simulink model "PLL_Simulering"  (R2020a)
settings: Solver=VariableStepAuto  StartTime=0  StopTime=0.5  RelTol=1e-3
InitFcn:
  | clear all;
libraries: powerlib x48, eePowerMeasurement x1, powerlib_meascontrol x1
(part 1 of 3)
settings Model: OrderedModelArguments=off  Creator=Bausa  LastModifiedBy=Bausa
settings SolverCC: AlgebraicLoopSolver=LineSearch
settings DataIOCC: ReturnWorkspaceOutputsName=tp1bad6c91_55d6_49eb_9d82_9787064f6320
settings OptimizationCC: DefaultParameterBehavior=Inlined  EnhancedBackFolding=on  PassReuseOutputArgsAs=Individual arguments  ZeroExternalMemoryAtStartup=off  ZeroInternalMemoryAtStartup=off  OptimizeBlockOrder=speed  DifferentSizesBufferReuse=on  OptimizationCustomize=off  EfficientTunableParamExpr=on
settings DebuggingCC: ParameterTunabilityLossMsg=error
settings SFSimCC: SimCustomHeaderCode="#include \"C_Functions.h\""  SimUserSources=C_Functions.c  MATLABDynamicMemAlloc=off
settings RTWCC: SystemTargetFile=ert.tlc  TemplateMakefile=ert_default_tmf
settings CodeAppCC: ForceParamTrailComments=on  IgnoreCustomStorageClasses=off  OperatorAnnotations=on  SimulinkDataObjDesc=on  SFDataObjDesc=on  InsertBlockDesc=on
settings ERTTargetCC: TargetLangStandard=C99 (ISO)  GenerateSampleERTMain=on  InlinedParameterPlacement=NonHierarchical  ERTCustomFileTemplate=example_file_process.tlc

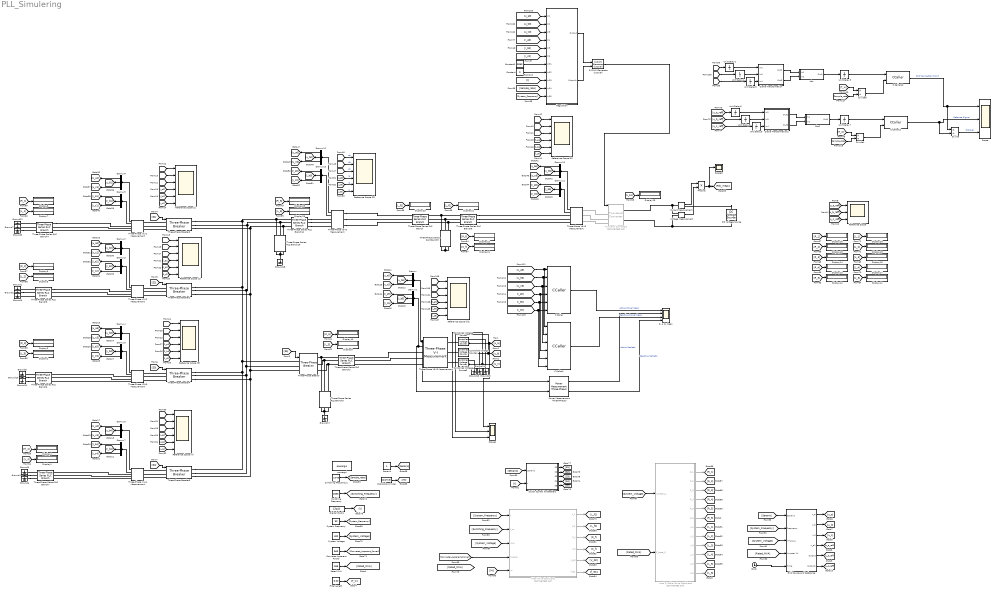
== system PLL_Simulering ==
  Abs : Subsystem
  Abs2 : Subsystem
  C Caller : CCaller  FunctionName=measure_P  PortSpecificationStruct="%)30     .    V L   8    (     @         %    \"     <    !     0         %  0 \"0    $    _    07)G3F%M90  4&]R=$YA;64 4V-O<&4     26YD97@     5'EP90      4VEZ90      27-';&]B86P   X    P    !@    @    $          4    (     0    ,    !         !   P!O=70 #@   #     &    \"     0         !0    @    !     P    $         $  # &]U=  .    .     8    (    !          %    \"     $    &     0         0   ...(+3703 chars)"
  C Caller1 : CCaller  FunctionName=measure_Q  PortSpecificationStruct="%)30     .    V L   8    (     @         %    \"     <    !     0         %  0 \"0    $    _    07)G3F%M90  4&]R=$YA;64 4V-O<&4     26YD97@     5'EP90      4VEZ90      27-';&]B86P   X    P    !@    @    $          4    (     0    ,    !         !   P!O=70 #@   #     &    \"     0         !0    @    !     P    $         $  # &]U=  .    .     8    (    !          %    \"     $    &     0         0   ...(+3703 chars)"
  C Caller10 : CCaller  FunctionName=MAF_Error_1  PortSpecificationStruct="%)30     .    : 4   8    (     @         %    \"     ,    !     0         %  0 \"0    $    _    07)G3F%M90  4&]R=$YA;64 4V-O<&4     26YD97@     5'EP90      4VEZ90      27-';&]B86P   X    P    !@    @    $          4    (     0    ,    !         !   P!O=70 #@   #     &    \"     0         !0    @    !     P    $         $  # &]U=  .    .     8    (    !          %    \"     $    &     0         0    !@   $]U='!U=   #@   #@    &    \"     8         !0    @    !     0    $         \"0    @               X    X    !@    @    $          4    (     0    8    !         !     &    9&]U8FQE   .    ,     8    (    !          %    \"     $    !     0         0  $ ,0    X    P    !@    @    ) @        4    (     0    $    !          (  0      #@   #@    &    \"     0         !0    @    !    !@    $         $     8   !S86UP;&4   X    X    !@    @    $          4    (     0    8    !         !     &    <V%M<&QE   .    .     8    (    !          %    \"     $    %     0         0    !0   $EN<'5T    #@   #@    &    \"     8         !0    @    !     0    $         \"0    @               X    X    !@    @    $          4    (     0    8    !         !     &    9&]U8FQE   .    ,     8    (    !          %    \"     $    !     0         0  $ ,0    X    P    !@    @    ) @        4    (     0    $    !          (  0      #@   #     &    \"     0         !0    @    !     P    $         $  # &QE;@ .    ,     8    (    !          %    \"     $    #     0         0  , ;&5N  X    X    !@    @    $          4    (     0    4    !         !     %    26YP=70    .    .     8    (    !@         %    \"     $    !     0         )    \"            / _#@   #@    &    \"     0         !0    @    !    !@    $         $     8   !U:6YT,S(   X    P    !@    @    $          4    (     0    $    !         !   0 Q    #@   #     &    \"     D\"        !0    @    !     0    $          @ !"
  C Caller12 : CCaller  FunctionName=MAF_Error_2  PortSpecificationStruct="%)30     .    : 4   8    (     @         %    \"     ,    !     0         %  0 \"0    $    _    07)G3F%M90  4&]R=$YA;64 4V-O<&4     26YD97@     5'EP90      4VEZ90      27-';&]B86P   X    P    !@    @    $          4    (     0    ,    !         !   P!O=70 #@   #     &    \"     0         !0    @    !     P    $         $  # &]U=  .    .     8    (    !          %    \"     $    &     0         0    !@   $]U='!U=   #@   #@    &    \"     8         !0    @    !     0    $         \"0    @               X    X    !@    @    $          4    (     0    8    !         !     &    9&]U8FQE   .    ,     8    (    !          %    \"     $    !     0         0  $ ,0    X    P    !@    @    ) @        4    (     0    $    !          (  0      #@   #@    &    \"     0         !0    @    !    !@    $         $     8   !S86UP;&4   X    X    !@    @    $          4    (     0    8    !         !     &    <V%M<&QE   .    .     8    (    !          %    \"     $    %     0         0    !0   $EN<'5T    #@   #@    &    \"     8         !0    @    !     0    $         \"0    @               X    X    !@    @    $          4    (     0    8    !         !     &    9&]U8FQE   .    ,     8    (    !          %    \"     $    !     0         0  $ ,0    X    P    !@    @    ) @        4    (     0    $    !          (  0      #@   #     &    \"     0         !0    @    !     P    $         $  # &QE;@ .    ,     8    (    !          %    \"     $    #     0         0  , ;&5N  X    X    !@    @    $          4    (     0    4    !         !     %    26YP=70    .    .     8    (    !@         %    \"     $    !     0         )    \"            / _#@   #@    &    \"     0         !0    @    !    !@    $         $     8   !U:6YT,S(   X    P    !@    @    $          4    (     0    $    !         !   0 Q    #@   #     &    \"     D\"        !0    @    !     0    $          @ !"
  Clarke Transformation : Subsystem
  Clarke Transformation2 : Subsystem
  Clock : Clock
  Constant : Constant  Value=0
  Constant1 : Constant  Value=50e3
  Controlled Voltage Source : powerlib/Electrical Sources/Controlled Voltage Source  Initialize=off  Source_Type=AC  Amplitude=0  Phase=0  Frequency=0  Measurements=None
  Controlled Voltage Source1 : powerlib/Electrical Sources/Controlled Voltage Source  Initialize=off  Source_Type=AC  Amplitude=0  Phase=0  Frequency=0  Measurements=None
  Controlled Voltage Source2 : powerlib/Electrical Sources/Controlled Voltage Source  Initialize=off  Source_Type=AC  Amplitude=0  Phase=0  Frequency=0  Measurements=None
  Converter Apparent Power : Constant  Value=5e3
  Current Measurement : powerlib/Measurements/Current Measurement  PhasorSimulation=off  OutputType=Complex  PSBequivalent=0
  DC Voltage Source : powerlib/Electrical Sources/DC Voltage Source  Amplitude=400  Measurements=None
  Demux{,1..13} (14 alike) : Demux  Outputs=3
  Digital Clock1 : DigitalClock
  Display{1..25,28..29} (27 alike) : Display
      Display1 settings: Format=short_e
      Display21 settings: Format=short_e
      Display23 settings: Format=short_e
      Display24 settings: Format=short_e
      Display25 settings: Format=short_e
      Display29 settings: Format=short_e
      Display5 settings: Format=short_e
      Display7 settings: Format=short_e
      Display9 settings: Format=short_e
  Divide : Product  Inputs=*/
  Divide1 : Product  Inputs=*/  OutDataTypeStr=uint32
  Divide3 : Product  Inputs=*/  OutDataTypeStr=uint32
  Filter Length : Constant  Value=0.02
  Filter Value Coeficients : MATLAB Function  Commented=on  TreatAsAtomicUnit=on
  Grid Source and Referance : Subsystem
  Ground{1..15,17..18} (17 alike) : powerlib/Elements/Ground  LConnTagsString=a
  Load & Cable Value Coeficients : MATLAB Function  Commented=on  TreatAsAtomicUnit=on
  Modulations Index : Constant  Value=2/sqrt(3)
  P- & Q- Meas. : Scope  NumInputPorts=4
  Power Measurement (Three-Phase) : eePowerMeasurement/Power Measurement (Three-Phase)  LabelModeActiveChoice=Continuous  F=60  K=[0]  Seq=Positive  Ts=0
      settings: SourceProductBaseCode=PS
  Product : Product
  Rated MVA : Constant  Value=2e6
  Referance Scope : Scope  NumInputPorts=3
  Referance Scope [0] : Scope  NumInputPorts=6
  Referance Scope [0]1 : Scope  NumInputPorts=6
  Referance Scope [1] : Scope  NumInputPorts=6
  Referance Scope [2] : Scope  NumInputPorts=6
  Referance Scope [3] : Scope  NumInputPorts=6
  Referance Scope [4] : Scope  NumInputPorts=6
  Referance Scope [6] : Scope  NumInputPorts=6
  Regulation : Subsystem
  SVPWM Generator (2-Level) : powerlib_meascontrol/Pulse & Signal Generators/SVPWM Generator (2-Level)  InputType=alpha-beta components  SwitchingPattern=Pattern #1  Fc=3000  ParUref=[0.8 0 50]  Ts=1e-6
      settings: SourceProductBaseCode=PS
  Scope : Scope  NumInputPorts=3
  Scope1 : Scope  NumInputPorts=3
  Scope3 : Scope
  Senario : Constant
  Switch Control for Breakers : MATLAB Function  TreatAsAtomicUnit=on
  Switching Frequency : Constant  Value=15e3
  Switching Frequency2 : Constant  Value=1e-06  OutDataTypeStr=double
  System Frequency : Constant  Value=50
  System Voltage : Constant  Value=400
  Three-Phase Series RLC Branch : powerlib/Elements/Three-Phase Series RLC Branch  LConnTagsString=A|B|C  RConnTagsString=A|B|C  BranchType=L  Resistance=1  Inductance=1.8e-3  Capacitance=1e-6  Measurements=None
  Three-Phase Series RLC Branch10 : powerlib/Elements/Three-Phase Series RLC Branch  LConnTagsString=A|B|C  RConnTagsString=A|B|C  BranchType=R  Resistance=1e9  Inductance=1e-3  Capacitance=1e-6  Measurements=None
  Three-Phase Series RLC Branch11 : powerlib/Elements/Three-Phase Series RLC Branch  LConnTagsString=A|B|C  RConnTagsString=A|B|C  BranchType=RL  Resistance=0.008268  Inductance=7.9572e-2  Capacitance=1e-6  Measurements=None
  Three-Phase Series RLC Branch2 : powerlib/Elements/Three-Phase Series RLC Branch  LConnTagsString=A|B|C  RConnTagsString=A|B|C  BranchType=RL  Resistance=0.005968  Inductance=1.9e-5  Capacitance=1e-6  Measurements=None
  Three-Phase Series RLC Branch3 : powerlib/Elements/Three-Phase Series RLC Branch  LConnTagsString=A|B|C  RConnTagsString=A|B|C  BranchType=R  Resistance=1e9  Inductance=1e-3  Capacitance=1e-6  Measurements=None
  Three-Phase Series RLC Branch{4..7} (4 alike) : powerlib/Elements/Three-Phase Series RLC Branch  LConnTagsString=A|B|C  RConnTagsString=A|B|C  BranchType=RL  Resistance=0.005968  Inductance=1.9e-4  Capacitance=1e-6  Measurements=None
  Three-Phase Series RLC Branch8 : powerlib/Elements/Three-Phase Series RLC Branch  LConnTagsString=A|B|C  RConnTagsString=A|B|C  BranchType=L  Resistance=1  Inductance=3e-4  Capacitance=1e-6  Measurements=None
  Three-Phase Series RLC Branch9 : powerlib/Elements/Three-Phase Series RLC Branch  LConnTagsString=A|B|C  RConnTagsString=A|B|C  BranchType=RC  Resistance=1e-6  Inductance=1e-3  Capacitance=25e-3  Measurements=None
  Three-Phase V0-I0 Measurement : powerlib/Measurements/Three-Phase V-I Measurement  VoltageMeasurement=phase-to-ground  SetLabelV=off  LabelV=Vabc  Vpu=off  VpuLL=off  CurrentMeasurement=yes  SetLabelI=off  LabelI=Iabc  Ipu=off  Pbase=100e6  Vbase=500e3  OutputType=Complex  PhasorSimulation=off  PSBequivalent=0
  Three-Phase V1-I1 Measurement : powerlib/Measurements/Three-Phase V-I Measurement  VoltageMeasurement=phase-to-ground  SetLabelV=off  LabelV=Vabc  Vpu=off  VpuLL=off  CurrentMeasurement=yes  SetLabelI=off  LabelI=Iabc  Ipu=off  Pbase=100e6  Vbase=500e3  OutputType=Complex  PhasorSimulation=off  PSBequivalent=0
  Three-Phase V2-I2 Measurement : powerlib/Measurements/Three-Phase V-I Measurement  VoltageMeasurement=phase-to-ground  SetLabelV=off  LabelV=Vabc  Vpu=off  VpuLL=off  CurrentMeasurement=yes  SetLabelI=off  LabelI=Iabc  Ipu=off  Pbase=100e6  Vbase=500e3  OutputType=Complex  PhasorSimulation=off  PSBequivalent=0
  Three-Phase V3-I3 Measurement : powerlib/Measurements/Three-Phase V-I Measurement  VoltageMeasurement=phase-to-ground  SetLabelV=off  LabelV=Vabc  Vpu=off  VpuLL=off  CurrentMeasurement=yes  SetLabelI=off  LabelI=Iabc  Ipu=off  Pbase=100e6  Vbase=500e3  OutputType=Complex  PhasorSimulation=off  PSBequivalent=0
  Three-Phase V4-I4 Measurement : powerlib/Measurements/Three-Phase V-I Measurement  VoltageMeasurement=phase-to-ground  SetLabelV=off  LabelV=Vabc  Vpu=off  VpuLL=off  CurrentMeasurement=yes  SetLabelI=off  LabelI=Iabc  Ipu=off  Pbase=100e6  Vbase=500e3  OutputType=Complex  PhasorSimulation=off  PSBequivalent=0
  Three-Phase V5-I5 Measurement : powerlib/Measurements/Three-Phase V-I Measurement  VoltageMeasurement=phase-to-ground  SetLabelV=off  LabelV=Vabc  Vpu=off  VpuLL=off  CurrentMeasurement=yes  SetLabelI=off  LabelI=Iabc  Ipu=off  Pbase=100e6  Vbase=500e3  OutputType=Complex  PhasorSimulation=off  PSBequivalent=0
  Three-Phase V6-I6 Measurement : powerlib/Measurements/Three-Phase V-I Measurement  VoltageMeasurement=phase-to-ground  SetLabelV=off  LabelV=Vabc  Vpu=off  VpuLL=off  CurrentMeasurement=yes  SetLabelI=off  LabelI=Iabc  Ipu=off  Pbase=100e6  Vbase=500e3  OutputType=Complex  PhasorSimulation=off  PSBequivalent=0
  Three-Phase Breaker : powerlib/Elements/Three-Phase Breaker  InitialState=open  SwitchA=on  SwitchB=on  SwitchC=on  SwitchTimes=9999  External=on  BreakerResistance=0.00001  SnubberResistance=1e9  SnubberCapacitance=0  Measurements=None
  Three-Phase Breaker{1..4} (4 alike) : powerlib/Elements/Three-Phase Breaker  InitialState=open  SwitchA=on  SwitchB=on  SwitchC=on  SwitchTimes="[1/60  5/60]"  External=on  BreakerResistance=0.01  SnubberResistance=1e6  SnubberCapacitance=inf  Measurements=None
  Two-Level Converter1 : powerlib/Power Electronics/Two-Level Converter  Commented=on  ModelType=Switching devices  Ron=1e-6  Rs=1e6  Cs=inf  Vforward=[0,0]  Ron_Diode=1e-3  Rs_Diode=1e6  Cs_Diode=inf  Vf_Diode=1e-3  Rs_CurrentSource=inf
      settings: SourceProductBaseCode=PS
  Unit Delay{2..9} (8 alike) : UnitDelay  SampleTime=-1  HasFrameUpgradeWarning=on
  Voltage Measurement : powerlib/Measurements/Voltage Measurement  PhasorSimulation=off  OutputType=Complex  PSBequivalent=0
  powergui : powerlib/powergui  Priority=1  SimulationMode=Discrete  SampleTime=1e-6  frequency=60  Iterations=50  frequencyindice=0  Pbase=100e6  ErrMax=1e-4  UnitsV=kV  UnitsW=MW  buscounter=0  FunctionMessages=off  echomessages=off  EnableUseOfTLC=off  CurrentSourceSwitches=off  DisableSnubberDevices=off  DisableRonSwitches=off  DisableVfSwitches=off  DisplayEquations=off  AutomaticDiscreteSolvers=off  SolverType=Tustin/Backward Euler (TBE)  Interpol=off  ExternalGateDelay=off  methode=off  Ts=100  x0status=blocks  SPID=on  SwTol=0  HookPort=off  NonlinearTolerance=1e-4  nMaxIteration=100  ContinueOnMaxIteration=off  RestoreLinks=warning  ResistiveCurrentMeasurement=off  Frange=[0:2:500]  Ylog=off  Xlog=on  ShowGrid=off  save=off  variable=ZData  structure=0  ZoomFFT=off  StartTime=0.0  cycles=1  DisplayStyle=1  fundamental=60  FreqAxis=off  MaxFrequency=1000  frequencyindicesteady=1  RmsSteady=1  display=off
  wires:
  Grid Source and Referance/1(u_a) -> [u_a]
  Grid Source and Referance/2(u_b) -> [u_b]
  Grid Source and Referance/3(u_c) -> [u_c]
  [u_a] -> Controlled Voltage Source/1, Scope1/1
  [u_c] -> Scope1/3, Controlled Voltage Source2/1
  [u_b] -> Scope1/2, Controlled Voltage Source1/1
  [S1] -> Three-Phase Breaker2/1
  [S2] -> Three-Phase Breaker1/1
  [S3] -> Three-Phase Breaker4/1
  [S4] -> Three-Phase Breaker3/1
  Three-Phase V5-I5 Measurement/1 -> Power Measurement (Three-Phase)/1, Demux/1
  Three-Phase V5-I5 Measurement/2 -> Power Measurement (Three-Phase)/2, Demux1/1
  [u_a_reff] -> Referance Scope/1
  [u_b_reff] -> Referance Scope/2
  [u_c_reff] -> Referance Scope/3
  Demux/1 -> [u_a5]
  Demux/2 -> [u_b5]
  Demux/3 -> [u_c5]
  Demux1/3 -> [i_c5]
  Demux1/1 -> [i_a5]
  Demux1/2 -> [i_b5]
  Demux6/1 -> [u_a4]
  Demux7/1 -> [i_a4]
  Demux7/3 -> [i_c4]
  Demux7/2 -> [i_b4]
  Demux6/2 -> [u_b4]
  Three-Phase V4-I4 Measurement/1 -> Demux6/1
  Demux6/3 -> [u_c4]
  Three-Phase V4-I4 Measurement/2 -> Demux7/1
  Demux4/1 -> [u_a3]
  Demux5/1 -> [i_a3]
  Demux5/3 -> [i_c3]
  Demux5/2 -> [i_b3]
  Demux4/2 -> [u_b3]
  Three-Phase V3-I3 Measurement/1 -> Demux4/1
  Demux4/3 -> [u_c3]
  Three-Phase V3-I3 Measurement/2 -> Demux5/1
  Demux2/1 -> [u_a2]
  Demux3/1 -> [i_a2]
  Demux3/3 -> [i_c2]
  Demux3/2 -> [i_b2]
  Demux2/2 -> [u_b2]
  Three-Phase V2-I2 Measurement/1 -> Demux2/1
  Demux2/3 -> [u_c2]
  Three-Phase V2-I2 Measurement/2 -> Demux3/1
  Demux8/1 -> [u_a1]
  Demux9/1 -> [i_a1]
  Demux9/3 -> [i_c1]
  Demux9/2 -> [i_b1]
  Demux8/2 -> [u_b1]
  Three-Phase V1-I1 Measurement/1 -> Demux8/1
  Demux8/3 -> [u_c1]
  Three-Phase V1-I1 Measurement/2 -> Demux9/1
  Demux10/2 -> [u_b6]
  Demux10/1 -> [u_a6]
  Demux11/1 -> [i_a6]
  Demux11/2 -> [i_b6]
  Demux11/3 -> [i_c6]
  Three-Phase V6-I6 Measurement/2 -> Demux11/1
  Demux10/3 -> [u_c6]
  Three-Phase V6-I6 Measurement/1 -> Demux10/1
  [u_c1] -> Referance Scope [1]/3
  [u_b1] -> Referance Scope [1]/2
  [u_a1] -> Referance Scope [1]/1
  [i_a1] -> Referance Scope [1]/4
  [i_b1] -> Referance Scope [1]/5
  [i_c1] -> Referance Scope [1]/6
  [i_b2] -> Referance Scope [2]/5
  [i_a2] -> Referance Scope [2]/4
  [i_c2] -> Referance Scope [2]/6
  [u_b2] -> Referance Scope [2]/2
  [u_c2] -> Referance Scope [2]/3
  [u_a2] -> Referance Scope [2]/1
  [i_b3] -> Referance Scope [3]/5
  [i_a3] -> Referance Scope [3]/4
  [i_c3] -> Referance Scope [3]/6
  [u_b3] -> Referance Scope [3]/2
  [u_c3] -> Referance Scope [3]/3
  [u_a3] -> Referance Scope [3]/1
  [i_b4] -> Referance Scope [4]/5
  [i_a4] -> Referance Scope [4]/4
  [i_c4] -> Referance Scope [4]/6
  [u_b4] -> Referance Scope [4]/2
  [u_c4] -> Referance Scope [4]/3
  [u_a4] -> Referance Scope [4]/1
  [i_b6] -> Referance Scope [6]/5
  [i_a6] -> Referance Scope [6]/4
  [i_c6] -> Referance Scope [6]/6
  [u_b6] -> Referance Scope [6]/2
  [u_c6] -> Referance Scope [6]/3
  [u_a6] -> Referance Scope [6]/1
  Demux12/2 -> [u_b0]
  Demux13/3 -> [i_c0]
  Demux12/3 -> [u_c0]
  Demux12/1 -> [u_a0]
  Demux13/1 -> [i_a0]
  Demux13/2 -> [i_b0]
  Three-Phase V0-I0 Measurement/1 -> Demux12/1
  Three-Phase V0-I0 Measurement/2 -> Demux13/1
  [u_b0] -> Referance Scope [0]/2  "Ub"
  [u_c0] -> Referance Scope [0]/3  "Uc"
  [i_c0] -> Referance Scope [0]/6  "Ic"
  [u_a0] -> Referance Scope [0]/1  "Ua"
  [i_a0] -> Referance Scope [0]/4  "Ia"
  [i_b0] -> Referance Scope [0]/5  "Ib"
  Grid Source and Referance/6(Output1) -> [u_c_reff]
  Grid Source and Referance/5(Output) -> [u_b_reff]
  Grid Source and Referance/4(u_a1) -> [u_a_reff]
  [R_4] -> Display4/1
  [L_4] -> Display1/1
  [R_3] -> Display3/1
  [L_3] -> Display2/1
  [R_2] -> Display6/1
  [L_2] -> Display5/1
  [R_1] -> Display8/1
  [L_1] -> Display7/1
  [R_5] -> Display10/1
  [L_5] -> Display9/1
  [R_5] -> Display12/1
  [R_3] -> Display14/1
  [R_4] -> Display13/1
  [R_1] -> Display16/1
  [R_2] -> Display15/1
  [L_4] -> Display17/1
  [L_3] -> Display18/1
  [L_1] -> Display20/1
  [L_2] -> Display19/1
  [L_5] -> Display11/1
  Divide/1 -> Scope/3  "Risidual"
  SVPWM Generator (2-Level)/1 -> Two-Level Converter1/1
  Switching Frequency/1 -> [Switching_Frequency]
  System Voltage/1 -> [System_Voltage]
  Senario/1 -> [Senario]
  Converter Apparent Power/1 -> [Converter_Apparent_Power]
  System Frequency/1 -> [System_Frequency]
  Switch Control for Breakers/1(S1) -> [S1]
  Switch Control for Breakers/5(S5) -> [S5]
  Switch Control for Breakers/2(S2) -> [S2]
  [t] -> Switch Control for Breakers/2(t)
  Switch Control for Breakers/3(S3) -> [S3]
  Switch Control for Breakers/4(S4) -> [S4]
  [Senario] -> Switch Control for Breakers/1(senario)
  Digital Clock1/1 -> [t]
  [System_Frequency] -> Filter Value Coeficients/1(f)
  [Switching_Frequency] -> Filter Value Coeficients/2(f_sw)
  Filter Value Coeficients/2(L_2) -> [L_f2]
  Filter Value Coeficients/1(L_1) -> [L_f1]
  Filter Value Coeficients/6(f_res) -> [f_res]
  [Mi] -> Filter Value Coeficients/5(Mi)
  Filter Value Coeficients/5(V_DC) -> [V_DC]
  Filter Value Coeficients/3(R_f) -> [R_f]
  [System_Voltage] -> Filter Value Coeficients/3(U_LL)
  Filter Value Coeficients/4(C_f) -> [C_f]
  Modulations Index/1 -> [Mi]
  Load & Cable Value Coeficients/3(R_3) -> [R_3]
  Load & Cable Value Coeficients/2(R_2) -> [R_2]
  Load & Cable Value Coeficients/4(R_4) -> [R_4]
  [System_Voltage] -> Load & Cable Value Coeficients/1(V_base_LL)
  Load & Cable Value Coeficients/11(L_5) -> [L_5]
  Load & Cable Value Coeficients/10(L_4) -> [L_4]
  Load & Cable Value Coeficients/9(L_3) -> [L_3]
  [Rated_MVA] -> Load & Cable Value Coeficients/2(S_base_3)
  Load & Cable Value Coeficients/8(L_2) -> [L_2]
  Load & Cable Value Coeficients/5(R_5) -> [R_5]
  Load & Cable Value Coeficients/7(L_1) -> [L_1]
  Load & Cable Value Coeficients/1(R_1) -> [R_1]
  Clock/1 -> Grid Source and Referance/5(Time)
  [Rated_MVA] -> Grid Source and Referance/4(Inverter VA)
  [System_Voltage] -> Grid Source and Referance/3(init_U_LL)
  [System_Frequency] -> Grid Source and Referance/2(Frequency)
  [Senario] -> Grid Source and Referance/1(Senario)
  [R_f] -> Display22/1
  [L_f1] -> Display21/1
  [L_f2] -> Display23/1
  [C_f] -> Display24/1
  [V_DC] -> Display25/1
  Rated MVA/1 -> [Rated_MVA]
  Load & Cable Value Coeficients/6(R_6) -> [R_6]
  Load & Cable Value Coeficients/12(L_6) -> [L_6]
  [i_a5] -> Referance Scope [0]1/4
  [i_b5] -> Referance Scope [0]1/5
  [i_c5] -> Referance Scope [0]1/6
  [u_a5] -> Referance Scope [0]1/1
  [u_b5] -> Referance Scope [0]1/2
  [u_c5] -> Referance Scope [0]1/3
  Clarke Transformation/1(Out2) -> Abs/1(In1)
  Clarke Transformation/2(Out3) -> Abs/2(In2)
  Filter Length/1 -> [T_w]
  Switching Frequency2/1 -> [Sample_rate]
  [Sample_rate] -> Divide3/2
  [T_w] -> Divide3/1
  C Caller10/1 -> Scope/1, Divide/1  "Grid Connection Point"
  Divide3/1 -> C Caller10/2
  Unit Delay3/1 -> C Caller10/1
  Abs/1(Out1) -> Unit Delay3/1
  [u_a0] -> Unit Delay2/1
  Unit Delay2/1 -> Clarke Transformation/1(In2)
  [u_b0] -> Unit Delay4/1
  Unit Delay4/1 -> Clarke Transformation/2(In3)
  Unit Delay5/1 -> Clarke Transformation/3(In4)
  [u_c0] -> Unit Delay5/1
  [u_b_reff] -> Unit Delay8/1
  Abs2/1(Out1) -> Unit Delay7/1
  [u_a_reff] -> Unit Delay6/1
  Unit Delay8/1 -> Clarke Transformation2/2(In3)
  Divide1/1 -> C Caller12/2
  Clarke Transformation2/2(Out3) -> Abs2/2(In2)
  C Caller12/1 -> Divide/2, Scope/2  "Refrance Signal"
  [T_w] -> Divide1/1
  [u_c_reff] -> Unit Delay9/1
  [Sample_rate] -> Divide1/2
  Unit Delay6/1 -> Clarke Transformation2/1(In2)
  Unit Delay9/1 -> Clarke Transformation2/3(In4)
  Clarke Transformation2/1(Out2) -> Abs2/1(In1)
  Unit Delay7/1 -> C Caller12/1
  [R_6] -> Display28/1
  [L_6] -> Display29/1
  [Converter_Apparent_Power] -> Filter Value Coeficients/4(S_base)
  Current Measurement/1 -> Product/1
  Voltage Measurement/1 -> Product/2
  Product/1 -> Scope3/1, [Pdc_meas]
  [S5] -> Three-Phase Breaker/1
  [Sample_rate] -> Regulation/10(In34)
  Constant/1 -> Regulation/8(In32)
  Constant1/1 -> Regulation/7(In31)
  [i_c0] -> Regulation/6(In6)
  [i_b0] -> Regulation/5(In5)
  [u_c0] -> Regulation/3(In3)
  [u_a0] -> Regulation/1(In1)
  Regulation/1(Output) -> SVPWM Generator (2-Level)/1
  Regulation/2(Output1) -> SVPWM Generator (2-Level)/2
  [t] -> Regulation/9(In33)
  [System_Frequency] -> Regulation/11(In35)
  [i_a0] -> Regulation/4(In4)
  [u_b0] -> Regulation/2(In2)
  [u_a5] -> C Caller1/1, C Caller/1
  [u_b5] -> C Caller1/2, C Caller/2
  [u_c5] -> C Caller1/3, C Caller/3
  [i_a5] -> C Caller1/4, C Caller/4
  [i_b5] -> C Caller1/5, C Caller/5
  [i_c5] -> C Caller1/6, C Caller/6
  C Caller/1 -> P- & Q- Meas./1  "Active Power Meas."
  C Caller1/1 -> P- & Q- Meas./3  "Reactive Power Meas."
  Power Measurement (Three-Phase)/1 -> P- & Q- Meas./2  "Active Matlabs"
  Power Measurement (Three-Phase)/2 -> P- & Q- Meas./4  "Reactive Matlabs"
  connections:
  Controlled Voltage Source/RConn1 -- Three-Phase V5-I5 Measurement/LConn1
  Controlled Voltage Source1/RConn1 -- Three-Phase V5-I5 Measurement/LConn2
  Controlled Voltage Source2/RConn1 -- Three-Phase V5-I5 Measurement/LConn3
  Three-Phase Breaker4/RConn1 -- Three-Phase Breaker3/RConn1 -- Three-Phase Series RLC Branch10/LConn1 -- Three-Phase Series RLC Branch11/LConn1 -- Three-Phase Breaker2/RConn1 -- Three-Phase Breaker1/RConn1 -- Three-Phase Breaker/LConn1
  DC Voltage Source/LConn1 -- Voltage Measurement/LConn2 -- Two-Level Converter1/RConn2
  Three-Phase Breaker2/LConn3 -- Three-Phase V1-I1 Measurement/LConn3
  Three-Phase Series RLC Branch4/RConn1 -- Three-Phase V1-I1 Measurement/RConn1
  Three-Phase V1-I1 Measurement/RConn3 -- Three-Phase Series RLC Branch4/RConn3
  Three-Phase Breaker2/LConn1 -- Three-Phase V1-I1 Measurement/LConn1
  Three-Phase Breaker2/LConn2 -- Three-Phase V1-I1 Measurement/LConn2
  Three-Phase V0-I0 Measurement/LConn3 -- Three-Phase Series RLC Branch/LConn3
  Two-Level Converter1/LConn1 -- Three-Phase V6-I6 Measurement/LConn1
  Two-Level Converter1/LConn2 -- Three-Phase V6-I6 Measurement/LConn2
  Three-Phase Series RLC Branch4/LConn1 -- Ground12/LConn1
  Ground8/LConn1 -- Three-Phase Series RLC Branch4/LConn3
  Two-Level Converter1/LConn3 -- Three-Phase V6-I6 Measurement/LConn3
  Three-Phase Breaker1/LConn1 -- Three-Phase V2-I2 Measurement/LConn1
  Three-Phase Breaker1/LConn3 -- Three-Phase V2-I2 Measurement/LConn3
  Three-Phase Breaker1/LConn2 -- Three-Phase V2-I2 Measurement/LConn2
  Three-Phase Breaker4/LConn1 -- Three-Phase V3-I3 Measurement/LConn1
  Three-Phase Breaker4/LConn2 -- Three-Phase V3-I3 Measurement/LConn2
  Three-Phase Breaker4/LConn3 -- Three-Phase V3-I3 Measurement/LConn3
  Three-Phase Breaker3/LConn3 -- Three-Phase V4-I4 Measurement/LConn3
  Three-Phase Breaker3/LConn1 -- Three-Phase V4-I4 Measurement/LConn1
  Three-Phase Breaker3/LConn2 -- Three-Phase V4-I4 Measurement/LConn2
  Ground15/LConn1 -- Controlled Voltage Source/LConn1
  Ground14/LConn1 -- Controlled Voltage Source1/LConn1
  Ground13/LConn1 -- Controlled Voltage Source2/LConn1
  Three-Phase Breaker4/RConn2 -- Three-Phase Breaker3/RConn2 -- Three-Phase Series RLC Branch10/LConn2 -- Three-Phase Series RLC Branch11/LConn2 -- Three-Phase Breaker2/RConn2 -- Three-Phase Breaker1/RConn2 -- Three-Phase Breaker/LConn2
  Three-Phase Breaker4/RConn3 -- Three-Phase Breaker3/RConn3 -- Three-Phase Breaker/LConn3 -- Three-Phase Series RLC Branch11/LConn3 -- Three-Phase Series RLC Branch10/LConn3 -- Three-Phase Breaker2/RConn3 -- Three-Phase Breaker1/RConn3
  Three-Phase Series RLC Branch2/LConn3 -- Three-Phase Series RLC Branch3/LConn3 -- Three-Phase Breaker/RConn3
  Three-Phase Series RLC Branch5/LConn3 -- Ground3/LConn1
  Three-Phase V2-I2 Measurement/RConn3 -- Three-Phase Series RLC Branch5/RConn3
  Three-Phase Series RLC Branch5/LConn1 -- Ground1/LConn1
  Three-Phase Series RLC Branch5/RConn1 -- Three-Phase V2-I2 Measurement/RConn1
  Ground11/LConn1 -- Three-Phase Series RLC Branch6/LConn3
  Three-Phase V3-I3 Measurement/RConn2 -- Three-Phase Series RLC Branch6/RConn2
  Three-Phase V3-I3 Measurement/RConn3 -- Three-Phase Series RLC Branch6/RConn3
  Three-Phase Series RLC Branch6/LConn1 -- Ground5/LConn1
  Three-Phase V3-I3 Measurement/RConn1 -- Three-Phase Series RLC Branch6/RConn1
  Three-Phase V0-I0 Measurement/LConn2 -- Three-Phase Series RLC Branch/LConn2
  Three-Phase Series RLC Branch2/LConn2 -- Three-Phase Series RLC Branch3/LConn2 -- Three-Phase Breaker/RConn2
  Ground17/LConn1 -- Three-Phase Series RLC Branch3/RConn1 -- Three-Phase Series RLC Branch3/RConn2 -- Three-Phase Series RLC Branch3/RConn3
  Three-Phase V5-I5 Measurement/RConn1 -- Three-Phase Series RLC Branch2/RConn1
  Three-Phase V5-I5 Measurement/RConn2 -- Three-Phase Series RLC Branch2/RConn2
  Three-Phase V5-I5 Measurement/RConn3 -- Three-Phase Series RLC Branch2/RConn3
  Three-Phase Series RLC Branch2/LConn1 -- Three-Phase Series RLC Branch3/LConn1 -- Three-Phase Breaker/RConn1
  Three-Phase V1-I1 Measurement/RConn2 -- Three-Phase Series RLC Branch4/RConn2
  Three-Phase Series RLC Branch4/LConn2 -- Ground7/LConn1
  Three-Phase V2-I2 Measurement/RConn2 -- Three-Phase Series RLC Branch5/RConn2
  Ground2/LConn1 -- Three-Phase Series RLC Branch5/LConn2
  Ground10/LConn1 -- Three-Phase Series RLC Branch6/LConn2
  Ground6/LConn1 -- Three-Phase Series RLC Branch7/LConn3
  Three-Phase V4-I4 Measurement/RConn3 -- Three-Phase Series RLC Branch7/RConn3
  Ground4/LConn1 -- Three-Phase Series RLC Branch7/LConn2
  Three-Phase Series RLC Branch7/LConn1 -- Ground9/LConn1
  Three-Phase V4-I4 Measurement/RConn2 -- Three-Phase Series RLC Branch7/RConn2
  Three-Phase V4-I4 Measurement/RConn1 -- Three-Phase Series RLC Branch7/RConn1
  Three-Phase Series RLC Branch8/RConn1 -- Three-Phase V6-I6 Measurement/RConn1
  Three-Phase Series RLC Branch8/RConn2 -- Three-Phase V6-I6 Measurement/RConn2
  Three-Phase Series RLC Branch8/RConn3 -- Three-Phase V6-I6 Measurement/RConn3
  Three-Phase Series RLC Branch8/LConn1 -- Three-Phase Series RLC Branch9/LConn1 -- Three-Phase Series RLC Branch/RConn1
  Three-Phase Series RLC Branch8/LConn2 -- Three-Phase Series RLC Branch9/LConn2 -- Three-Phase Series RLC Branch/RConn2
  Three-Phase Series RLC Branch8/LConn3 -- Three-Phase Series RLC Branch9/LConn3 -- Three-Phase Series RLC Branch/RConn3
  Three-Phase Series RLC Branch9/RConn1 -- Three-Phase Series RLC Branch9/RConn3 -- Three-Phase Series RLC Branch9/RConn2
  Three-Phase V0-I0 Measurement/LConn1 -- Three-Phase Series RLC Branch/LConn1
  Three-Phase Series RLC Branch11/RConn1 -- Three-Phase V0-I0 Measurement/RConn1
  Three-Phase Series RLC Branch11/RConn2 -- Three-Phase V0-I0 Measurement/RConn2
  Three-Phase Series RLC Branch11/RConn3 -- Three-Phase V0-I0 Measurement/RConn3
  Three-Phase Series RLC Branch10/RConn2 -- Three-Phase Series RLC Branch10/RConn1 -- Ground18/LConn1 -- Three-Phase Series RLC Branch10/RConn3
  DC Voltage Source/RConn1 -- Current Measurement/RConn1
  Current Measurement/LConn1 -- Voltage Measurement/LConn1 -- Two-Level Converter1/RConn1

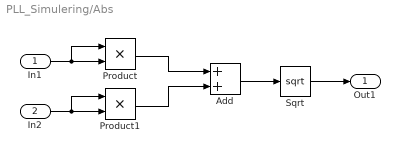
== system PLL_Simulering/Abs ==
  In1 : Inport
  In2 : Inport  Port=2
  Add : Sum  OutDataTypeStr=double
  Product : Product
  Product1 : Product  OutDataTypeStr=double
  Sqrt : Sqrt  OutDataTypeStr=double  SaturateOnIntegerOverflow=on
  Out1 : Outport
  wires:
  In1/1 -> Product/1, Product/2
  In2/1 -> Product1/1, Product1/2
  Product/1 -> Add/1
  Product1/1 -> Add/2
  Add/1 -> Sqrt/1
  Sqrt/1 -> Out1/1

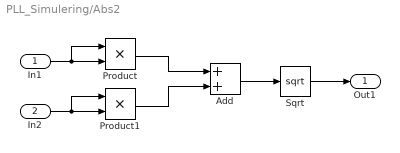
== system PLL_Simulering/Abs2 ==
  In1 : Inport
  In2 : Inport  Port=2
  Add : Sum  OutDataTypeStr=double
  Product : Product
  Product1 : Product  OutDataTypeStr=double
  Sqrt : Sqrt  OutDataTypeStr=double  SaturateOnIntegerOverflow=on
  Out1 : Outport
  wires:
  In1/1 -> Product/1, Product/2
  In2/1 -> Product1/1, Product1/2
  Product/1 -> Add/1
  Product1/1 -> Add/2
  Add/1 -> Sqrt/1
  Sqrt/1 -> Out1/1

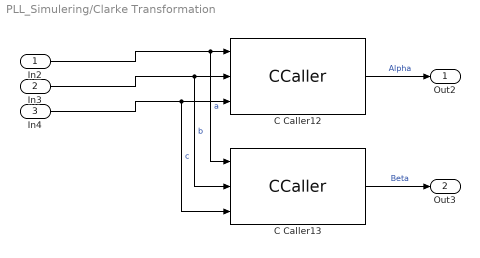
== system PLL_Simulering/Clarke Transformation ==
  In2 : Inport
  In3 : Inport  Port=2
  In4 : Inport  Port=3
  C Caller12 : CCaller  FunctionName=Clarke_alpha  PortSpecificationStruct="%)30     .    ^ 8   8    (     @         %    \"     0    !     0         %  0 \"0    $    _    07)G3F%M90  4&]R=$YA;64 4V-O<&4     26YD97@     5'EP90      4VEZ90      27-';&]B86P   X    P    !@    @    $          4    (     0    ,    !         !   P!O=70 #@   #     &    \"     0         !0    @    !     P    $         $  # &]U=  .    .     8    (    !          %    \"     $    &     0         0   ...(+2020 chars)"
  C Caller13 : CCaller  FunctionName=Clarke_beta  PortSpecificationStruct="%)30     .    ^ 8   8    (     @         %    \"     0    !     0         %  0 \"0    $    _    07)G3F%M90  4&]R=$YA;64 4V-O<&4     26YD97@     5'EP90      4VEZ90      27-';&]B86P   X    P    !@    @    $          4    (     0    ,    !         !   P!O=70 #@   #     &    \"     0         !0    @    !     P    $         $  # &]U=  .    .     8    (    !          %    \"     $    &     0         0   ...(+2020 chars)"
  Out2 : Outport
  Out3 : Outport  Port=2
  wires:
  In2/1 -> C Caller13/1, C Caller12/1  "a"
  In3/1 -> C Caller13/2, C Caller12/2  "b"
  In4/1 -> C Caller13/3, C Caller12/3  "c"
  C Caller12/1 -> Out2/1  "Alpha"
  C Caller13/1 -> Out3/1  "Beta"

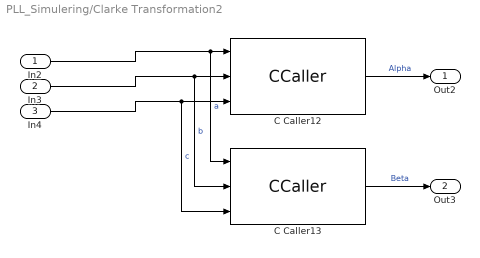
== system PLL_Simulering/Clarke Transformation2 ==
  In2 : Inport
  In3 : Inport  Port=2
  In4 : Inport  Port=3
  C Caller12 : CCaller  FunctionName=Clarke_alpha  PortSpecificationStruct="%)30     .    ^ 8   8    (     @         %    \"     0    !     0         %  0 \"0    $    _    07)G3F%M90  4&]R=$YA;64 4V-O<&4     26YD97@     5'EP90      4VEZ90      27-';&]B86P   X    P    !@    @    $          4    (     0    ,    !         !   P!O=70 #@   #     &    \"     0         !0    @    !     P    $         $  # &]U=  .    .     8    (    !          %    \"     $    &     0         0   ...(+2020 chars)"
  C Caller13 : CCaller  FunctionName=Clarke_beta  PortSpecificationStruct="%)30     .    ^ 8   8    (     @         %    \"     0    !     0         %  0 \"0    $    _    07)G3F%M90  4&]R=$YA;64 4V-O<&4     26YD97@     5'EP90      4VEZ90      27-';&]B86P   X    P    !@    @    $          4    (     0    ,    !         !   P!O=70 #@   #     &    \"     0         !0    @    !     P    $         $  # &]U=  .    .     8    (    !          %    \"     $    &     0         0   ...(+2020 chars)"
  Out2 : Outport
  Out3 : Outport  Port=2
  wires:
  In2/1 -> C Caller13/1, C Caller12/1  "a"
  In3/1 -> C Caller13/2, C Caller12/2  "b"
  In4/1 -> C Caller13/3, C Caller12/3  "c"
  C Caller12/1 -> Out2/1  "Alpha"
  C Caller13/1 -> Out3/1  "Beta"
